simulink model "EvitarObstaculo"  (R2019a)
settings: Solver=ode3  StartTime=0.0  StopTime=100.0  FixedStep=Ts  RelTol=1e-3
values from neighbouring files (symbols this model uses):
  obsx = 1    [TrajectoryControl.m]
  obsy = 0    [TrajectoryControl.m]
  th_0 = 0    [TrajectoryControl.m]
  Ts = 100e-3    (= 0.1)    [TrajectoryControl.m]
  x_0 = 0.2    [TrajectoryControl.m]
  y_0 = 0    [TrajectoryControl.m]
undefined symbols (not defined in the file or in its folder): DiscIntNeverNeededParam, sigbuilder_block
libraries: fuzblock x1, simulink x1
settings Model: PacingRate=0.028000  Creator=Alex  LastModifiedBy=Alex
settings DataIOCC: ReturnWorkspaceOutputs=off

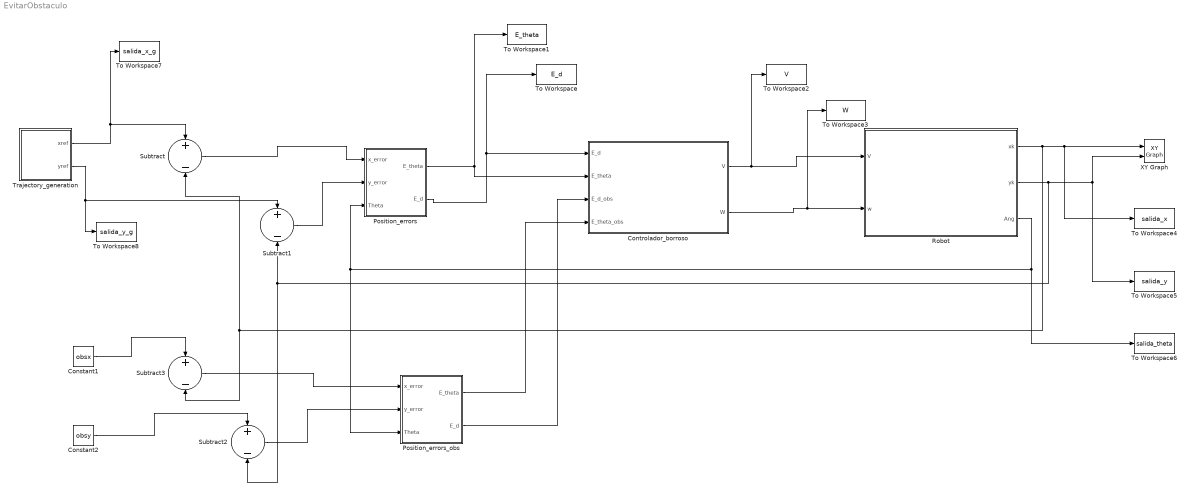
== system EvitarObstaculo ==
  Constant1 : Constant  Value=obsx
  Constant2 : Constant  Value=obsy
  Controlador_borroso : Subsystem
  Position_errors : Subsystem
  Position_errors_obs : Subsystem
  "Robot " : Subsystem
  Subtract{,1..3} (4 alike) : Sum  Inputs=+-
  To Workspace : ToWorkspace  VariableName=E_d  SaveFormat=Structure With Time  SampleTime=-1
  To Workspace1 : ToWorkspace  VariableName=E_theta  SaveFormat=Structure With Time  SampleTime=-1
  To Workspace2 : ToWorkspace  VariableName=V  SaveFormat=Structure With Time  SampleTime=-1
  To Workspace3 : ToWorkspace  VariableName=W  SaveFormat=Structure With Time  SampleTime=-1
  To Workspace4 : ToWorkspace  VariableName=salida_x  SaveFormat=Structure With Time  SampleTime=-1
  To Workspace5 : ToWorkspace  VariableName=salida_y  SaveFormat=Structure With Time  SampleTime=-1
  To Workspace6 : ToWorkspace  VariableName=salida_theta  SaveFormat=Structure With Time  SampleTime=-1
  To Workspace7 : ToWorkspace  VariableName=salida_x_g  SaveFormat=Structure With Time  SampleTime=-1
  To Workspace8 : ToWorkspace  VariableName=salida_y_g  SaveFormat=Structure With Time  SampleTime=-1
  Trajectory_generation : Subsystem
  XY Graph : simulink/Sinks/XY Graph  xmin=-5  xmax=5  ymin=-5  ymax=5  st=-1
  wires:
  Subtract/1 -> Position_errors/1("x_error ")
  Subtract1/1 -> Position_errors/2("y_error ")
  "Robot "/1(xk) -> Subtract/2, Subtract3/2, To Workspace4/1, XY Graph/1
  "Robot "/2(yk) -> Subtract2/2, Subtract1/2, To Workspace5/1, XY Graph/2
  "Robot "/3(Ang) -> Position_errors_obs/3(Theta), Position_errors/3(Theta), To Workspace6/1
  Position_errors/2(E_d) -> Controlador_borroso/1(E_d), To Workspace/1
  Position_errors/1(E_theta) -> Controlador_borroso/2(E_theta), To Workspace1/1
  Trajectory_generation/1(xref) -> Subtract/1, To Workspace7/1
  Trajectory_generation/2(yref) -> Subtract1/1, To Workspace8/1
  Constant1/1 -> Subtract3/1
  Constant2/1 -> Subtract2/1
  Subtract3/1 -> Position_errors_obs/1("x_error ")
  Subtract2/1 -> Position_errors_obs/2("y_error ")
  Controlador_borroso/1(V) -> "Robot "/1(V), To Workspace2/1
  Controlador_borroso/2(W) -> To Workspace3/1, "Robot "/2("w ")
  Position_errors_obs/1(E_theta) -> Controlador_borroso/4(E_theta_obs)
  Position_errors_obs/2(E_d) -> Controlador_borroso/3(E_d_obs)

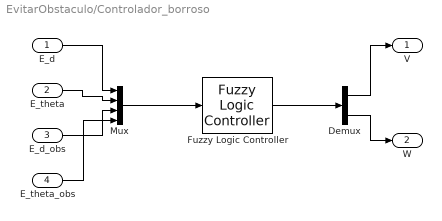
== system EvitarObstaculo/Controlador_borroso ==
  E_d : Inport
  E_theta : Inport  Port=2
  E_d_obs : Inport  Port=3
  E_theta_obs : Inport  Port=4
  Demux : Demux  Outputs=2
  Fuzzy Logic Controller : fuzblock/Fuzzy Logic  Controller  FIS='Controlador2.fis'  OutputSampleNumber=101  DataType=double  FuzzifiedInputs=off  RuleFiringStrengths=off  RuleOutputs=off  AggregatedOutputs=off  SimulateUsing=Interpreted execution  OutOfRangeInputValueMessage=warning  NoRuleFiredMessage=warning  EmptyOutputFuzzySetMessage=warning
  Mux : Mux
  V : Outport
  W : Outport  Port=2
  wires:
  Fuzzy Logic Controller/1 -> Demux/1
  Demux/1 -> V/1
  Mux/1 -> Fuzzy Logic Controller/1
  E_d/1 -> Mux/1
  E_d_obs/1 -> Mux/3
  Demux/2 -> W/1
  E_theta/1 -> Mux/2
  E_theta_obs/1 -> Mux/4

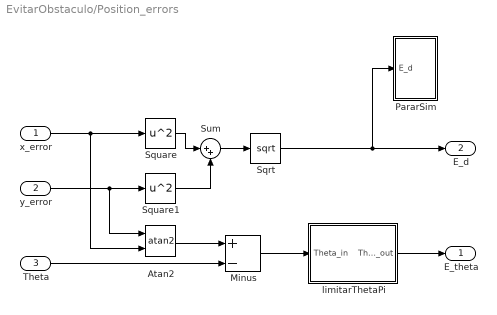
== system EvitarObstaculo/Position_errors ==
  "x_error " : Inport
  "y_error " : Inport  Port=2
  Theta : Inport  Port=3
  Atan2 : Trigonometry  Operator=atan2
  Minus : Sum  Inputs=+-
  PararSim : Subsystem
  Sqrt : Sqrt  SaturateOnIntegerOverflow=on
  Square : Math  Operator=square  SaturateOnIntegerOverflow=on
  Square1 : Math  Operator=square  SaturateOnIntegerOverflow=on
  Sum : Sum  Inputs=|++
  limitarThetaPi : Subsystem
  E_theta : Outport  VectorParamsAs1DForOutWhenUnconnected=on
  E_d : Outport  Port=2  VectorParamsAs1DForOutWhenUnconnected=on
  wires:
  "x_error "/1 -> Square/1, Atan2/2
  "y_error "/1 -> Atan2/1, Square1/1
  Theta/1 -> Minus/2
  Sum/1 -> Sqrt/1
  Sqrt/1 -> PararSim/1("E_d "), E_d/1
  Square/1 -> Sum/1
  Square1/1 -> Sum/2
  Atan2/1 -> Minus/1
  Minus/1 -> limitarThetaPi/1(Theta_in)
  limitarThetaPi/1(Theta_out) -> E_theta/1

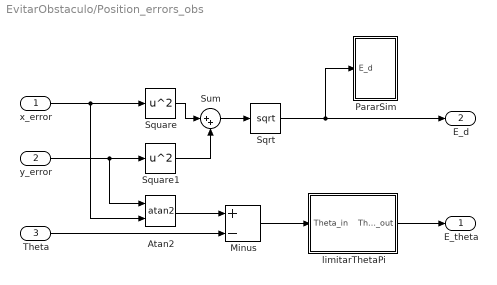
== system EvitarObstaculo/Position_errors_obs ==
  "x_error " : Inport
  "y_error " : Inport  Port=2
  Theta : Inport  Port=3
  Atan2 : Trigonometry  Operator=atan2
  Minus : Sum  Inputs=+-
  PararSim : Subsystem
  Sqrt : Sqrt  SaturateOnIntegerOverflow=on
  Square : Math  Operator=square  SaturateOnIntegerOverflow=on
  Square1 : Math  Operator=square  SaturateOnIntegerOverflow=on
  Sum : Sum  Inputs=|++
  limitarThetaPi : Subsystem
  E_theta : Outport  VectorParamsAs1DForOutWhenUnconnected=on
  E_d : Outport  Port=2  VectorParamsAs1DForOutWhenUnconnected=on
  wires:
  "x_error "/1 -> Square/1, Atan2/2
  "y_error "/1 -> Atan2/1, Square1/1
  Theta/1 -> Minus/2
  Sum/1 -> Sqrt/1
  Sqrt/1 -> PararSim/1("E_d "), E_d/1
  Square/1 -> Sum/1
  Square1/1 -> Sum/2
  Atan2/1 -> Minus/1
  Minus/1 -> limitarThetaPi/1(Theta_in)
  limitarThetaPi/1(Theta_out) -> E_theta/1

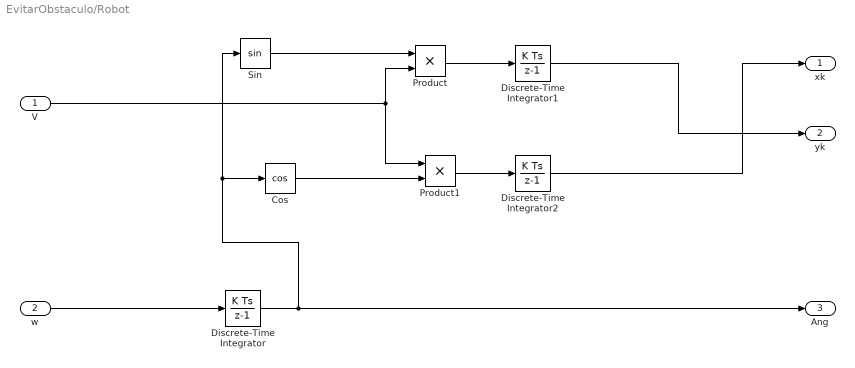
== system EvitarObstaculo/Robot  ==
  V : Inport
  "w " : Inport  Port=2
  Cos : Trigonometry  Operator=cos
  Discrete-Time Integrator : DiscreteIntegrator  SampleTime=-1  ICPrevOutput=DiscIntNeverNeededParam  ICPrevScaledInput=DiscIntNeverNeededParam
  Discrete-Time Integrator1 : DiscreteIntegrator  SampleTime=-1  ICPrevOutput=DiscIntNeverNeededParam  ICPrevScaledInput=DiscIntNeverNeededParam
  Discrete-Time Integrator2 : DiscreteIntegrator  SampleTime=-1  ICPrevOutput=DiscIntNeverNeededParam  ICPrevScaledInput=DiscIntNeverNeededParam
  Product : Product
  Product1 : Product
  Sin : Trigonometry
  xk : Outport
  yk : Outport  Port=2
  Ang : Outport  Port=3
  wires:
  Sin/1 -> Product/1
  Cos/1 -> Product1/2
  V/1 -> Product1/1, Product/2
  Product/1 -> Discrete-Time Integrator1/1
  Discrete-Time Integrator2/1 -> xk/1
  Discrete-Time Integrator1/1 -> yk/1
  Product1/1 -> Discrete-Time Integrator2/1
  "w "/1 -> Discrete-Time Integrator/1
  Discrete-Time Integrator/1 -> Ang/1, Cos/1, Sin/1

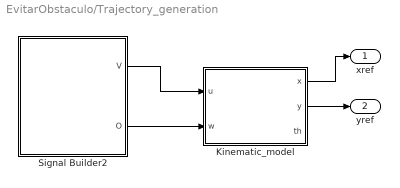
== system EvitarObstaculo/Trajectory_generation ==
  Kinematic_model : Subsystem
  Signal Builder2 : Subsystem  Tag=STV Subsys  LoadFcn=sigbuilder_block('load');  StartFcn=sigbuilder_block('start');  StopFcn=sigbuilder_block('stop');  ClipboardFcn=sigbuilder_block('clipboard');  mask(Sigbuilder block){tuvar=[0:10]}
      mask help: Sigbuilder GUI
      mask init:
      | if ~strcmp(get_param(bdroot(gcbh),'SimulationStatus'),'stopped') tuvar = sigbuilder_block('maskInit'); end
      settings: CopyFcn=sigbuilder_block('copy');  DeleteFcn=sigbuilder_block('delete');  ModelCloseFcn=sigbuilder_block('modelClose');  PreSaveFcn=sigbuilder_block('preSave');  PauseFcn=sigbuilder_block('pause')  ContinueFcn=sigbuilder_block('continue')  NameChangeFcn=sigbuilder_block('namechange');  OpenFcn=sigbuilder_block('open',[60 82.4 534.4 508 ]);  CloseFcn=sigbuilder_block('close');
      mask Display: plot(0, 0, 100, 100,[2, 2, 32, 32, 2], [68, 8, 8, 68, 68],[32, 2], [38, 38], [32, 19, 2],[53, 60, 44], [32, 17, 17, 2],[16, 16, 31, 31]);txt = getActiveGroup(gcbh);text(2, 100, txt,'verticalAlignment', 'top');
  xref : Outport
  yref : Outport  Port=2
  wires:
  Signal Builder2/1(V) -> Kinematic_model/1(u)
  Signal Builder2/2(O) -> Kinematic_model/2(w)
  Kinematic_model/1(x) -> xref/1
  Kinematic_model/2(y) -> yref/1

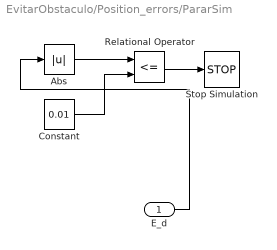
== system EvitarObstaculo/Position_errors/PararSim ==
  "E_d " : Inport
  Abs : Abs
  Constant : Constant  Value=0.01
  Relational Operator : RelationalOperator  Operator=<=  OutDataTypeStr=boolean  RndMeth=Simplest
  Stop Simulation : Stop
  wires:
  Abs/1 -> Relational Operator/1
  Constant/1 -> Relational Operator/2
  "E_d "/1 -> Abs/1
  Relational Operator/1 -> Stop Simulation/1

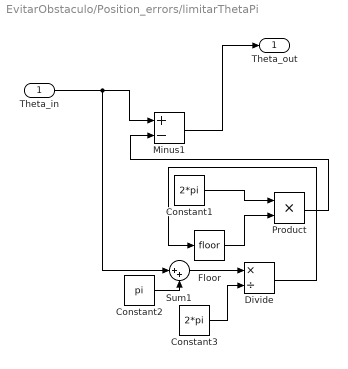
== system EvitarObstaculo/Position_errors/limitarThetaPi ==
  Theta_in : Inport
  Constant1 : Constant  Value=2*pi
  Constant2 : Constant  Value=pi
  Constant3 : Constant  Value=2*pi
  Divide : Product  Inputs=*/
  Floor : Rounding
  Minus1 : Sum  Inputs=+-
  Product : Product
  Sum1 : Sum  Inputs=|++
  Theta_out : Outport
  wires:
  Constant1/1 -> Product/1
  Theta_in/1 -> Sum1/1, Minus1/1
  Sum1/1 -> Divide/1
  Floor/1 -> Product/2
  Minus1/1 -> Theta_out/1
  Constant2/1 -> Sum1/2
  Divide/1 -> Floor/1
  Product/1 -> Minus1/2
  Constant3/1 -> Divide/2

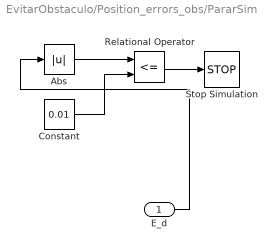
== system EvitarObstaculo/Position_errors_obs/PararSim ==
  "E_d " : Inport
  Abs : Abs
  Constant : Constant  Value=0.01
  Relational Operator : RelationalOperator  Operator=<=  OutDataTypeStr=boolean  RndMeth=Simplest
  Stop Simulation : Stop
  wires:
  Abs/1 -> Relational Operator/1
  Constant/1 -> Relational Operator/2
  "E_d "/1 -> Abs/1
  Relational Operator/1 -> Stop Simulation/1

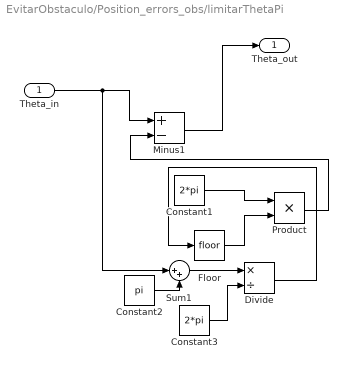
== system EvitarObstaculo/Position_errors_obs/limitarThetaPi ==
  Theta_in : Inport
  Constant1 : Constant  Value=2*pi
  Constant2 : Constant  Value=pi
  Constant3 : Constant  Value=2*pi
  Divide : Product  Inputs=*/
  Floor : Rounding
  Minus1 : Sum  Inputs=+-
  Product : Product
  Sum1 : Sum  Inputs=|++
  Theta_out : Outport
  wires:
  Constant1/1 -> Product/1
  Theta_in/1 -> Sum1/1, Minus1/1
  Sum1/1 -> Divide/1
  Floor/1 -> Product/2
  Minus1/1 -> Theta_out/1
  Constant2/1 -> Sum1/2
  Divide/1 -> Floor/1
  Product/1 -> Minus1/2
  Constant3/1 -> Divide/2

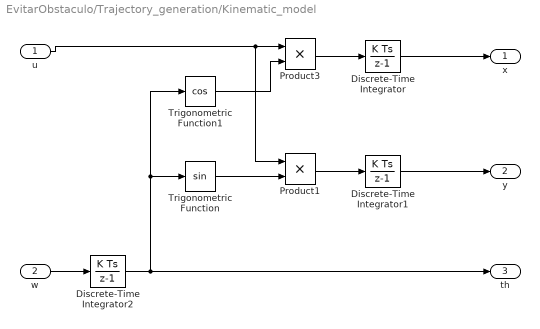
== system EvitarObstaculo/Trajectory_generation/Kinematic_model ==
  u : Inport
  w : Inport  Port=2
  Discrete-Time Integrator : DiscreteIntegrator  InitialCondition=x_0  SampleTime=Ts  ICPrevOutput=DiscIntNeverNeededParam  ICPrevScaledInput=DiscIntNeverNeededParam
  Discrete-Time Integrator1 : DiscreteIntegrator  InitialCondition=y_0  SampleTime=Ts  ICPrevOutput=DiscIntNeverNeededParam  ICPrevScaledInput=DiscIntNeverNeededParam
  Discrete-Time Integrator2 : DiscreteIntegrator  InitialCondition=th_0  SampleTime=Ts  ICPrevOutput=DiscIntNeverNeededParam  ICPrevScaledInput=DiscIntNeverNeededParam
  Product1 : Product
  Product3 : Product
  Trigonometric Function : Trigonometry
  Trigonometric Function1 : Trigonometry  Operator=cos
  x : Outport
  y : Outport  Port=2
  th : Outport  Port=3
  wires:
  Discrete-Time Integrator2/1 -> Trigonometric Function1/1, Trigonometric Function/1, th/1
  Product1/1 -> Discrete-Time Integrator1/1
  Product3/1 -> Discrete-Time Integrator/1
  w/1 -> Discrete-Time Integrator2/1
  Trigonometric Function/1 -> Product1/2
  u/1 -> Product1/1, Product3/1
  Trigonometric Function1/1 -> Product3/2
  Discrete-Time Integrator1/1 -> y/1
  Discrete-Time Integrator/1 -> x/1

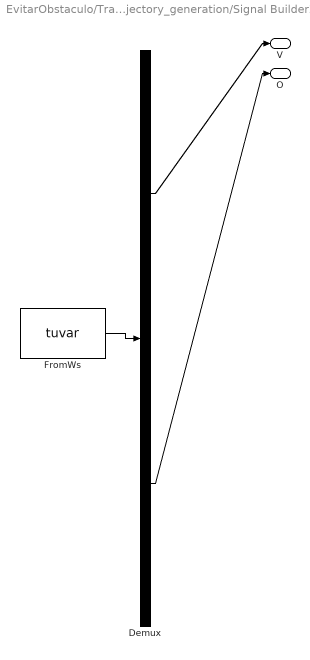
== system EvitarObstaculo/Trajectory_generation/Signal Builder2 ==
  Demux : Demux  Tag=STV Demux  Outputs=2
  FromWs : FromWorkspace  Tag=STV FromWs  VariableName=tuvar  SampleTime=0
      SigBuilderData=|
      | common.afterFinalStr = 'Extrapolate'
      | common.sampleTime = '0'
      | dataSet.timeRange = [0 115]
      | dataSet.name = 'Group 1'
      | sbobj.Groups.Name = 'Group 1'
      | sbobj.Groups.Signals(1).Name = 'V'
      | sbobj.Groups.Signals(1).XData = [0 87 87 115]
      | sbobj.Groups.Signals(1).YData = [0.25 0.25 0 0]
      | sbobj.Groups.Signals(2).Name = 'O'
      | sbobj.Groups.Signals(2).XData = [0 12 12 30.849 30.849 55.981 55.981 74.83 74.83 99.962 115]
      | sbobj.Groups.Signals(2).YData = [0 0 0.25 0.25 -0.25 -0.25 0.25 0.25 0 0 0]
      | sbobj.Groups.TimeRange = [0 115]
  V : Outport  Tag=STV Outport
  O : Outport  Tag=STV Outport  Port=2
  wires:
  FromWs/1 -> Demux/1
  Demux/1 -> V/1
  Demux/2 -> O/1
